simulink model "Ejemplo_6"  (R2013a)
settings: Solver=ode45  StartTime=0.0  StopTime=10.0  RelTol=1e-3
libraries: simulink x1
settings Model: Creator=Miguel  LastModifiedBy=Miguel
settings DataIOCC: LimitDataPoints=off

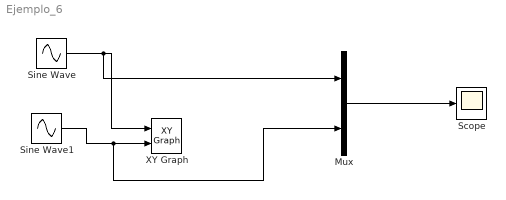
== system Ejemplo_6 ==
  Mux : Mux  Inputs=2
  Scope : Scope
      settings: TickLabels=on  ShowLegends=on
  Sine Wave : Sin  SampleTime=0
  Sine Wave1 : Sin  Frequency=2  Phase=pi/4  SampleTime=0
  XY Graph : simulink/Sinks/XY Graph  xmin=-1  xmax=1  ymin=-1  ymax=1  st=-1
  wires:
  Mux/1 -> Scope/1
  Sine Wave/1 -> Mux/1, XY Graph/1
  Sine Wave1/1 -> Mux/2, XY Graph/2
